simulink model "Three_Tank_V1"  (R2019a)
settings: Solver=VariableStepAuto  StartTime=0.0  StopTime=10.0  RelTol=1e-3
settings Model: DataDictionary=Three_Tank_V1.sldd  OrderedModelArguments=off  Creator=rdkluijv  LastModifiedBy=rdkluijv

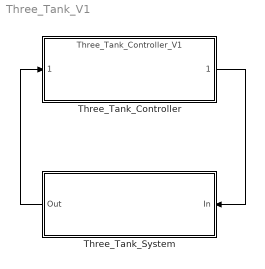
== system Three_Tank_V1 ==
  Three_Tank_Controller : ModelReference  ModelNameDialog=Three_Tank_Controller_V1.slx  SimulationMode=Normal  ModelReferenceVersion=1.4
  Three_Tank_System : Subsystem  Variant=on
  wires:
  Three_Tank_Controller/1 -> Three_Tank_System/1(In)
  Three_Tank_System/1(Out) -> Three_Tank_Controller/1

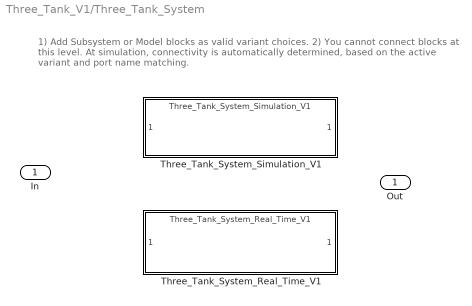
== system Three_Tank_V1/Three_Tank_System ==
  note: 1) Add Subsystem or Model blocks as valid variant choices.
      | 2) You cannot connect blocks at this level. At simulation, connectivity is automatically
      | determined, based on the active variant and port name matching.
  In : Inport  OutDataTypeStr=Bus: Bus_COSI
  Three_Tank_System_Real_Time_V1 : ModelReference  ModelNameDialog=Three_Tank_System_Real_Time_V1.slx  VariantControl=V_REAL_TIME  ModelReferenceVersion=1.4
  Three_Tank_System_Simulation_V1 : ModelReference  DisableCoverage=on  ModelNameDialog=Three_Tank_System_Simulation_V1.slx  VariantControl=V_SIMULATION  ModelReferenceVersion=1.5
  Out : Outport  OutDataTypeStr=Bus: Bus_CISO
